simulink library "MedusaPremix"  (R2022b)
settings: Solver=VariableStepAuto  StartTime=0.0  StopTime=10.0  RelTol=1e-3
values from neighbouring files (symbols this model uses):
  PremixConfig = struct('sample_rate_in_hertz', sample_rate_in_hertz,                            'frame_size', frame_size,                            'rgain_SILENT_GAIN', rgain_SILENT_GAIN,                            'granularity', internal_granularity,                            'LR_in', LR_in, 'LR_out', LR_out,                            'CS_in', CS_in, 'CS_out', CS_out,                            'NumCenterOut' ...(+550 chars)    [MedusaPremixInit.m]
  PremixTune = MedusaPremixTuneInit(tuneFileName, headrestTuneFileName, overheadTuneFileName, MedusaParams)    [MedusaPremixInit.m]    (also in MedusaPremixTuneInit.m = load(tuneFileName))
undefined symbols (not defined in the file or in its folder): carModel, mode, MSConfig, Row
libraries: TuneVar x286, TOP x202, dspmtrx3 x146, FeaturePath x86, matrix_library x20, PooliirLib x8, Pooliir x4
(part 14 of 22)

== system MedusaPremix/PremixWithMonoSurround/Full Mixing Matrix_Center Surround/Surround Level Control/Ramper ==
  RTC Recv Trigger : Inport
  target gains (linear) : Inport  Port=2
  ramp rate : Inport  Port=3
  ramp time : Inport  Port=4
  check sequence trigger : Inport  Port=5
  Data Store Memory : DataStoreMemory  DataStoreName=Premix_Freeze_CS  ReadBeforeWriteMsg=warning  WriteAfterWriteMsg=warning  WriteAfterReadMsg=warning  ShowAdditionalParam=off  OutDataTypeStr=boolean
  Data Store Memory1 : DataStoreMemory  DataStoreName=Premix_frameCount_CS  ReadBeforeWriteMsg=warning  WriteAfterWriteMsg=warning  WriteAfterReadMsg=warning  InitialValue=zeros(MedusaPremixConfig.CS_out,MedusaPremixConfig.CS_in)  ShowAdditionalParam=off  OutDataTypeStr=int32
  Data Store Memory2 : DataStoreMemory  DataStoreName=Premix_rampCoeff_CS  ReadBeforeWriteMsg=warning  WriteAfterWriteMsg=warning  WriteAfterReadMsg=warning  InitialValue=ones(MedusaPremixConfig.CS_out,MedusaPremixConfig.CS_in)  ShowAdditionalParam=off  OutDataTypeStr=single
  check sequence : MATLAB Function  TreatAsAtomicUnit=on
  control : MATLAB Function  TreatAsAtomicUnit=on
  process : MATLAB Function  TreatAsAtomicUnit=on
  ramping done : Outport  VectorParamsAs1DForOutWhenUnconnected=off
  wires:
  target gains (linear)/1 -> control/1(target_gains_linear)
  RTC Recv Trigger/1 -> control/Trigger
  check sequence/1(done) -> ramping done/1
  check sequence trigger/1 -> check sequence/Trigger
  ramp rate/1 -> control/2(rampRate)
  ramp time/1 -> control/3(rampTime)

== system MedusaPremix/PremixWithMonoSurround/Full Mixing Matrix_Left/Fader Downmix/Fading Backward ==
  frontFadeGain : Inport
  backwardDownmixThreshold : Inport  Port=2
  backwardDownmixMax : Inport  Port=3
  Action Port : ActionPort
  Constant : Constant  OutDataTypeStr=single
  Divide : Product  Inputs=*/
  EPS : Constant  Value=eps('single')
  Max : MinMax  Function=max  Inputs=2
  Min : MinMax  Inputs=2
  Multiply : Product
  Subtract : Sum  Inputs=+-
  downmix : Outport  VectorParamsAs1DForOutWhenUnconnected=off
  wires:
  Multiply/1 -> downmix/1
  backwardDownmixMax/1 -> Multiply/2
  Subtract/1 -> Multiply/1
  Divide/1 -> Subtract/2
  Max/1 -> Divide/2
  Min/1 -> Divide/1  "minFadeGain"
  EPS/1 -> Max/2
  Constant/1 -> Subtract/1
  backwardDownmixThreshold/1 -> Max/1, Min/2
  frontFadeGain/1 -> Min/1

== system MedusaPremix/PremixWithMonoSurround/Full Mixing Matrix_Left/Fader Downmix/Fading Forward ==
  backFadeGain : Inport
  forwardDownmixThreshold : Inport  Port=2
  forwardDownmixMax : Inport  Port=3
  Action Port : ActionPort
  Constant : Constant  OutDataTypeStr=single
  Divide : Product  Inputs=*/
  EPS : Constant  Value=eps('single')
  Max : MinMax  Function=max  Inputs=2
  Min : MinMax  Inputs=2
  Multiply : Product
  Subtract : Sum  Inputs=+-
  downmix : Outport  VectorParamsAs1DForOutWhenUnconnected=off
  wires:
  Multiply/1 -> downmix/1
  forwardDownmixMax/1 -> Multiply/2
  Subtract/1 -> Multiply/1
  Divide/1 -> Subtract/2
  Max/1 -> Divide/2
  Min/1 -> Divide/1  "minFadeGain"
  EPS/1 -> Max/2
  Constant/1 -> Subtract/1
  forwardDownmixThreshold/1 -> Max/1, Min/2
  backFadeGain/1 -> Min/1

== system MedusaPremix/PremixWithMonoSurround/Full Mixing Matrix_Left/Surround Level Control/Ramper ==
  RTC Recv Trigger : Inport
  target gains (linear) : Inport  Port=2
  ramp rate : Inport  Port=3
  ramp time : Inport  Port=4
  check sequence trigger : Inport  Port=5
  Data Store Memory : DataStoreMemory  DataStoreName=Premix_Freeze_Left  ReadBeforeWriteMsg=warning  WriteAfterWriteMsg=warning  WriteAfterReadMsg=warning  ShowAdditionalParam=off  OutDataTypeStr=boolean
  Data Store Memory1 : DataStoreMemory  DataStoreName=Premix_frameCount_Left  ReadBeforeWriteMsg=warning  WriteAfterWriteMsg=warning  WriteAfterReadMsg=warning  InitialValue=zeros(MedusaPremixConfig.LR_out,MedusaPremixConfig.LR_in)  ShowAdditionalParam=off  OutDataTypeStr=int32
  Data Store Memory2 : DataStoreMemory  DataStoreName=Premix_rampCoeff_Left  ReadBeforeWriteMsg=warning  WriteAfterWriteMsg=warning  WriteAfterReadMsg=warning  InitialValue=ones(MedusaPremixConfig.LR_out,MedusaPremixConfig.LR_in)  ShowAdditionalParam=off  OutDataTypeStr=single
  check sequence : MATLAB Function  TreatAsAtomicUnit=on
  control : MATLAB Function  TreatAsAtomicUnit=on
  process : MATLAB Function  TreatAsAtomicUnit=on
  ramping done : Outport  VectorParamsAs1DForOutWhenUnconnected=off
  wires:
  target gains (linear)/1 -> control/1(target_gains_linear)
  RTC Recv Trigger/1 -> control/Trigger
  check sequence/1(done) -> ramping done/1
  check sequence trigger/1 -> check sequence/Trigger
  ramp time/1 -> control/3(rampTime)
  ramp rate/1 -> control/2(rampRate)

== system MedusaPremix/PremixWithMonoSurround/Full Mixing Matrix_Right/Fader Downmix/Fading Backward ==
  frontFadeGain : Inport
  backwardDownmixThreshold : Inport  Port=2
  backwardDownmixMax : Inport  Port=3
  Action Port : ActionPort
  Constant : Constant  OutDataTypeStr=single
  Divide : Product  Inputs=*/
  EPS : Constant  Value=eps('single')
  Max : MinMax  Function=max  Inputs=2
  Min : MinMax  Inputs=2
  Multiply : Product
  Subtract : Sum  Inputs=+-
  downmix : Outport  VectorParamsAs1DForOutWhenUnconnected=off
  wires:
  Multiply/1 -> downmix/1
  backwardDownmixMax/1 -> Multiply/2
  Subtract/1 -> Multiply/1
  Divide/1 -> Subtract/2
  Max/1 -> Divide/2
  Min/1 -> Divide/1  "minFadeGain"
  EPS/1 -> Max/2
  Constant/1 -> Subtract/1
  backwardDownmixThreshold/1 -> Max/1, Min/2
  frontFadeGain/1 -> Min/1

== system MedusaPremix/PremixWithMonoSurround/Full Mixing Matrix_Right/Fader Downmix/Fading Forward ==
  backFadeGain : Inport
  forwardDownmixThreshold : Inport  Port=2
  forwardDownmixMax : Inport  Port=3
  Action Port : ActionPort
  Constant : Constant  OutDataTypeStr=single
  Divide : Product  Inputs=*/
  EPS : Constant  Value=eps('single')
  Max : MinMax  Function=max  Inputs=2
  Min : MinMax  Inputs=2
  Multiply : Product
  Subtract : Sum  Inputs=+-
  downmix : Outport  VectorParamsAs1DForOutWhenUnconnected=off
  wires:
  Multiply/1 -> downmix/1
  forwardDownmixMax/1 -> Multiply/2
  Subtract/1 -> Multiply/1
  Divide/1 -> Subtract/2
  Max/1 -> Divide/2
  Min/1 -> Divide/1  "minFadeGain"
  EPS/1 -> Max/2
  Constant/1 -> Subtract/1
  forwardDownmixThreshold/1 -> Max/1, Min/2
  backFadeGain/1 -> Min/1

== system MedusaPremix/PremixWithMonoSurround/Full Mixing Matrix_Right/Surround Level Control/Ramper ==
  RTC Recv Trigger : Inport
  target gains (linear) : Inport  Port=2
  ramp rate : Inport  Port=3
  ramp time : Inport  Port=4
  check sequence trigger : Inport  Port=5
  Data Store Memory : DataStoreMemory  DataStoreName=Premix_Freeze_Right  ReadBeforeWriteMsg=warning  WriteAfterWriteMsg=warning  WriteAfterReadMsg=warning  ShowAdditionalParam=off  OutDataTypeStr=boolean
  Data Store Memory1 : DataStoreMemory  DataStoreName=Premix_frameCount_Right  ReadBeforeWriteMsg=warning  WriteAfterWriteMsg=warning  WriteAfterReadMsg=warning  InitialValue=zeros(MedusaPremixConfig.LR_out,MedusaPremixConfig.LR_in)  ShowAdditionalParam=off  OutDataTypeStr=int32
  Data Store Memory2 : DataStoreMemory  DataStoreName=Premix_rampCoeff_Right  ReadBeforeWriteMsg=warning  WriteAfterWriteMsg=warning  WriteAfterReadMsg=warning  InitialValue=ones(MedusaPremixConfig.LR_out,MedusaPremixConfig.LR_in)  ShowAdditionalParam=off  OutDataTypeStr=single
  check sequence : MATLAB Function  TreatAsAtomicUnit=on
  control : MATLAB Function  TreatAsAtomicUnit=on
  process : MATLAB Function  TreatAsAtomicUnit=on
  ramping done : Outport  VectorParamsAs1DForOutWhenUnconnected=off
  wires:
  target gains (linear)/1 -> control/1(target_gains_linear)
  RTC Recv Trigger/1 -> control/Trigger
  check sequence/1(done) -> ramping done/1
  check sequence trigger/1 -> check sequence/Trigger
  ramp rate/1 -> control/2(rampRate)
  ramp time/1 -> control/3(rampTime)

== system MedusaPremix/PremixWithMonoSurroundAndCae/CS Processing/Mono-Surround/Left Mixer ==
  AudioIn : Inport
  MixCoeff : Inport  Port=2
  Matrix Multiply1 : Product  Multiplication=Matrix(*)
  Transpose1 : Math  Operator=transpose  SignedPower=on
  Output : Outport  VectorParamsAs1DForOutWhenUnconnected=off
  wires:
  Transpose1/1 -> Matrix Multiply1/2
  MixCoeff/1 -> Transpose1/1
  AudioIn/1 -> Matrix Multiply1/1
  Matrix Multiply1/1 -> Output/1

== system MedusaPremix/PremixWithMonoSurroundAndCae/CS Processing/Mono-Surround/MS Tune ==
  TOP : TOP/TOP  TriggerInit=[260 -150 405 -90]  TopName=Phi  DataType=single  BankNumber=0  Role=Automatic
      settings: SourceProductName=Bose Talaria
  TOP1 : TOP/TOP  TriggerInit=[260 -70 405 -10]  TopName=CosPhi  DataType=single  BankNumber=0  Role=Automatic
      settings: SourceProductName=Bose Talaria
  TOP2 : TOP/TOP  TriggerInit=[260 10 405 70]  TopName=SinPhi  DataType=single  BankNumber=0  Role=Automatic
      settings: SourceProductName=Bose Talaria
  TranslateTrigger : TuneVar/TranslateTrigger  TriggerInit=[66 -245 104 -190]
      settings: SourceProductName=Bose Talaria
  Tune Variable : TuneVar/Tune Variable  TuneName=PhaseAngle  SpecifyMaxSize=off  VariableDim=1 (Row)  MaxSize=[1 1]  PackageName=mode  TunabilityNumber=1  MinValue=[]  MaxValue=[]  TriggerInit=[-270 -65 -100 -15]  MaskValue=MSConfig.DefaultPhaseAngle
      settings: SourceProductName=Bose Talaria
  translation : MATLAB Function  TreatAsAtomicUnit=on
  phi : Outport  VectorParamsAs1DForOutWhenUnconnected=off
  cos(phi) : Outport  Port=2  VectorParamsAs1DForOutWhenUnconnected=off
  sin(phi) : Outport  Port=3  VectorParamsAs1DForOutWhenUnconnected=off
  wires:
  TOP2/1 -> sin(phi)/1  "SinPhi"
  translation/3(sin_phi) -> TOP2/1
  TOP1/1 -> cos(phi)/1  "CosPhi"
  translation/2(cos_phi) -> TOP1/1
  Tune Variable/1 -> translation/1(PhaseAngle)  "PhaseAngle"
  TOP/1 -> phi/1  "Phi"
  TranslateTrigger/1 -> translation/Trigger
  translation/1(phi) -> TOP/1

== system MedusaPremix/PremixWithMonoSurroundAndCae/CS Processing/Mono-Surround/Right Mixer ==
  AudioIn : Inport
  MixCoeff : Inport  Port=2
  Matrix Multiply1 : Product  Multiplication=Matrix(*)
  Transpose1 : Math  Operator=transpose  SignedPower=on
  Output : Outport  VectorParamsAs1DForOutWhenUnconnected=off
  wires:
  Transpose1/1 -> Matrix Multiply1/2
  MixCoeff/1 -> Transpose1/1
  AudioIn/1 -> Matrix Multiply1/1
  Matrix Multiply1/1 -> Output/1

== system MedusaPremix/PremixWithMonoSurroundAndCae/CS Processing/Mono-Surround/SOS A ==
  AudioIn : Inport
  TuneIn : Inport  Port=2
  Hilbert SOS A : Subsystem  TreatAsAtomicUnit=on
  If : If  IfExpression=(u1==0) | (u1==180)
  Merge : Merge
  Pass-through : Subsystem  TreatAsAtomicUnit=on
  Out : Outport  VectorParamsAs1DForOutWhenUnconnected=off
  wires:
  Merge/1 -> Out/1
  Hilbert SOS A/1(Out) -> Merge/2
  Pass-through/1(Out1) -> Merge/1
  TuneIn/1 -> If/1
  If/2 -> Hilbert SOS A/Action
  If/1 -> Pass-through/Action
  AudioIn/1 -> Pass-through/1(In1), Hilbert SOS A/1(AudioIn)

== system MedusaPremix/PremixWithMonoSurroundAndCae/CS Processing/Mono-Surround/SOS B ==
  AudioIn : Inport
  TuneIn : Inport  Port=2
  Hilbert SOS B : Subsystem  TreatAsAtomicUnit=on
  If : If  IfExpression=(u1==0) | (u1==180)
  Merge : Merge
  Pass-through : Subsystem  TreatAsAtomicUnit=on
  Out : Outport  VectorParamsAs1DForOutWhenUnconnected=off
  wires:
  Merge/1 -> Out/1
  Hilbert SOS B/1(Out) -> Merge/2
  Pass-through/1(Out1) -> Merge/1
  TuneIn/1 -> If/1
  If/2 -> Hilbert SOS B/Action
  If/1 -> Pass-through/Action
  AudioIn/1 -> Pass-through/1(In1), Hilbert SOS B/1(AudioIn)

== system MedusaPremix/PremixWithMonoSurroundAndCae/Full Mixing Matrix_Center Surround/Fader Downmix/Fading Backward ==
  frontFadeGain : Inport
  backwardDownmixThreshold : Inport  Port=2
  backwardDownmixMax : Inport  Port=3
  Action Port : ActionPort
  Constant : Constant  OutDataTypeStr=single
  Divide : Product  Inputs=*/
  EPS : Constant  Value=eps('single')
  Max : MinMax  Function=max  Inputs=2
  Min : MinMax  Inputs=2
  Multiply : Product
  Subtract : Sum  Inputs=+-
  downmix : Outport  VectorParamsAs1DForOutWhenUnconnected=off
  wires:
  Multiply/1 -> downmix/1
  backwardDownmixMax/1 -> Multiply/2
  Subtract/1 -> Multiply/1
  Divide/1 -> Subtract/2
  Max/1 -> Divide/2
  Min/1 -> Divide/1  "minFadeGain"
  EPS/1 -> Max/2
  Constant/1 -> Subtract/1
  backwardDownmixThreshold/1 -> Max/1, Min/2
  frontFadeGain/1 -> Min/1

== system MedusaPremix/PremixWithMonoSurroundAndCae/Full Mixing Matrix_Center Surround/Fader Downmix/Fading Forward ==
  backFadeGain : Inport
  forwardDownmixThreshold : Inport  Port=2
  forwardDownmixMax : Inport  Port=3
  Action Port : ActionPort
  Constant : Constant  OutDataTypeStr=single
  Divide : Product  Inputs=*/
  EPS : Constant  Value=eps('single')
  Max : MinMax  Function=max  Inputs=2
  Min : MinMax  Inputs=2
  Multiply : Product
  Subtract : Sum  Inputs=+-
  downmix : Outport  VectorParamsAs1DForOutWhenUnconnected=off
  wires:
  Multiply/1 -> downmix/1
  forwardDownmixMax/1 -> Multiply/2
  Subtract/1 -> Multiply/1
  Divide/1 -> Subtract/2
  Max/1 -> Divide/2
  Min/1 -> Divide/1  "minFadeGain"
  EPS/1 -> Max/2
  Constant/1 -> Subtract/1
  forwardDownmixThreshold/1 -> Max/1, Min/2
  backFadeGain/1 -> Min/1

== system MedusaPremix/PremixWithMonoSurroundAndCae/Full Mixing Matrix_Center Surround/Surround Level Control/Ramper ==
  RTC Recv Trigger : Inport
  target gains (linear) : Inport  Port=2
  ramp rate : Inport  Port=3
  ramp time : Inport  Port=4
  check sequence trigger : Inport  Port=5
  Data Store Memory : DataStoreMemory  DataStoreName=Premix_Freeze_CS  ReadBeforeWriteMsg=warning  WriteAfterWriteMsg=warning  WriteAfterReadMsg=warning  ShowAdditionalParam=off  OutDataTypeStr=boolean
  Data Store Memory1 : DataStoreMemory  DataStoreName=Premix_frameCount_CS  ReadBeforeWriteMsg=warning  WriteAfterWriteMsg=warning  WriteAfterReadMsg=warning  InitialValue=zeros(MedusaPremixConfig.CS_out,MedusaPremixConfig.CS_in)  ShowAdditionalParam=off  OutDataTypeStr=int32
  Data Store Memory2 : DataStoreMemory  DataStoreName=Premix_rampCoeff_CS  ReadBeforeWriteMsg=warning  WriteAfterWriteMsg=warning  WriteAfterReadMsg=warning  InitialValue=ones(MedusaPremixConfig.CS_out,MedusaPremixConfig.CS_in)  ShowAdditionalParam=off  OutDataTypeStr=single
  check sequence : MATLAB Function  TreatAsAtomicUnit=on
  control : MATLAB Function  TreatAsAtomicUnit=on
  process : MATLAB Function  TreatAsAtomicUnit=on
  ramping done : Outport  VectorParamsAs1DForOutWhenUnconnected=off
  wires:
  target gains (linear)/1 -> control/1(target_gains_linear)
  RTC Recv Trigger/1 -> control/Trigger
  check sequence/1(done) -> ramping done/1
  check sequence trigger/1 -> check sequence/Trigger
  ramp rate/1 -> control/2(rampRate)
  ramp time/1 -> control/3(rampTime)

== system MedusaPremix/PremixWithMonoSurroundAndCae/Full Mixing Matrix_Left/Fader Downmix/Fading Backward ==
  frontFadeGain : Inport
  backwardDownmixThreshold : Inport  Port=2
  backwardDownmixMax : Inport  Port=3
  Action Port : ActionPort
  Constant : Constant  OutDataTypeStr=single
  Divide : Product  Inputs=*/
  EPS : Constant  Value=eps('single')
  Max : MinMax  Function=max  Inputs=2
  Min : MinMax  Inputs=2
  Multiply : Product
  Subtract : Sum  Inputs=+-
  downmix : Outport  VectorParamsAs1DForOutWhenUnconnected=off
  wires:
  Multiply/1 -> downmix/1
  backwardDownmixMax/1 -> Multiply/2
  Subtract/1 -> Multiply/1
  Divide/1 -> Subtract/2
  Max/1 -> Divide/2
  Min/1 -> Divide/1  "minFadeGain"
  EPS/1 -> Max/2
  Constant/1 -> Subtract/1
  backwardDownmixThreshold/1 -> Max/1, Min/2
  frontFadeGain/1 -> Min/1

== system MedusaPremix/PremixWithMonoSurroundAndCae/Full Mixing Matrix_Left/Fader Downmix/Fading Forward ==
  backFadeGain : Inport
  forwardDownmixThreshold : Inport  Port=2
  forwardDownmixMax : Inport  Port=3
  Action Port : ActionPort
  Constant : Constant  OutDataTypeStr=single
  Divide : Product  Inputs=*/
  EPS : Constant  Value=eps('single')
  Max : MinMax  Function=max  Inputs=2
  Min : MinMax  Inputs=2
  Multiply : Product
  Subtract : Sum  Inputs=+-
  downmix : Outport  VectorParamsAs1DForOutWhenUnconnected=off
  wires:
  Multiply/1 -> downmix/1
  forwardDownmixMax/1 -> Multiply/2
  Subtract/1 -> Multiply/1
  Divide/1 -> Subtract/2
  Max/1 -> Divide/2
  Min/1 -> Divide/1  "minFadeGain"
  EPS/1 -> Max/2
  Constant/1 -> Subtract/1
  forwardDownmixThreshold/1 -> Max/1, Min/2
  backFadeGain/1 -> Min/1

== system MedusaPremix/PremixWithMonoSurroundAndCae/Full Mixing Matrix_Left/Surround Level Control/Ramper ==
  RTC Recv Trigger : Inport
  target gains (linear) : Inport  Port=2
  ramp rate : Inport  Port=3
  ramp time : Inport  Port=4
  check sequence trigger : Inport  Port=5
  Data Store Memory : DataStoreMemory  DataStoreName=Premix_Freeze_Left  ReadBeforeWriteMsg=warning  WriteAfterWriteMsg=warning  WriteAfterReadMsg=warning  ShowAdditionalParam=off  OutDataTypeStr=boolean
  Data Store Memory1 : DataStoreMemory  DataStoreName=Premix_frameCount_Left  ReadBeforeWriteMsg=warning  WriteAfterWriteMsg=warning  WriteAfterReadMsg=warning  InitialValue=zeros(MedusaPremixConfig.LR_out,MedusaPremixConfig.LR_in)  ShowAdditionalParam=off  OutDataTypeStr=int32
  Data Store Memory2 : DataStoreMemory  DataStoreName=Premix_rampCoeff_Left  ReadBeforeWriteMsg=warning  WriteAfterWriteMsg=warning  WriteAfterReadMsg=warning  InitialValue=ones(MedusaPremixConfig.LR_out,MedusaPremixConfig.LR_in)  ShowAdditionalParam=off  OutDataTypeStr=single
  check sequence : MATLAB Function  TreatAsAtomicUnit=on
  control : MATLAB Function  TreatAsAtomicUnit=on
  process : MATLAB Function  TreatAsAtomicUnit=on
  ramping done : Outport  VectorParamsAs1DForOutWhenUnconnected=off
  wires:
  target gains (linear)/1 -> control/1(target_gains_linear)
  RTC Recv Trigger/1 -> control/Trigger
  check sequence/1(done) -> ramping done/1
  check sequence trigger/1 -> check sequence/Trigger
  ramp time/1 -> control/3(rampTime)
  ramp rate/1 -> control/2(rampRate)

== system MedusaPremix/PremixWithMonoSurroundAndCae/Full Mixing Matrix_Right/Fader Downmix/Fading Backward ==
  frontFadeGain : Inport
  backwardDownmixThreshold : Inport  Port=2
  backwardDownmixMax : Inport  Port=3
  Action Port : ActionPort
  Constant : Constant  OutDataTypeStr=single
  Divide : Product  Inputs=*/
  EPS : Constant  Value=eps('single')
  Max : MinMax  Function=max  Inputs=2
  Min : MinMax  Inputs=2
  Multiply : Product
  Subtract : Sum  Inputs=+-
  downmix : Outport  VectorParamsAs1DForOutWhenUnconnected=off
  wires:
  Multiply/1 -> downmix/1
  backwardDownmixMax/1 -> Multiply/2
  Subtract/1 -> Multiply/1
  Divide/1 -> Subtract/2
  Max/1 -> Divide/2
  Min/1 -> Divide/1  "minFadeGain"
  EPS/1 -> Max/2
  Constant/1 -> Subtract/1
  backwardDownmixThreshold/1 -> Max/1, Min/2
  frontFadeGain/1 -> Min/1

== system MedusaPremix/PremixWithMonoSurroundAndCae/Full Mixing Matrix_Right/Fader Downmix/Fading Forward ==
  backFadeGain : Inport
  forwardDownmixThreshold : Inport  Port=2
  forwardDownmixMax : Inport  Port=3
  Action Port : ActionPort
  Constant : Constant  OutDataTypeStr=single
  Divide : Product  Inputs=*/
  EPS : Constant  Value=eps('single')
  Max : MinMax  Function=max  Inputs=2
  Min : MinMax  Inputs=2
  Multiply : Product
  Subtract : Sum  Inputs=+-
  downmix : Outport  VectorParamsAs1DForOutWhenUnconnected=off
  wires:
  Multiply/1 -> downmix/1
  forwardDownmixMax/1 -> Multiply/2
  Subtract/1 -> Multiply/1
  Divide/1 -> Subtract/2
  Max/1 -> Divide/2
  Min/1 -> Divide/1  "minFadeGain"
  EPS/1 -> Max/2
  Constant/1 -> Subtract/1
  forwardDownmixThreshold/1 -> Max/1, Min/2
  backFadeGain/1 -> Min/1

== system MedusaPremix/PremixWithMonoSurroundAndCae/Full Mixing Matrix_Right/Surround Level Control/Ramper ==
  RTC Recv Trigger : Inport
  target gains (linear) : Inport  Port=2
  ramp rate : Inport  Port=3
  ramp time : Inport  Port=4
  check sequence trigger : Inport  Port=5
  Data Store Memory : DataStoreMemory  DataStoreName=Premix_Freeze_Right  ReadBeforeWriteMsg=warning  WriteAfterWriteMsg=warning  WriteAfterReadMsg=warning  ShowAdditionalParam=off  OutDataTypeStr=boolean
  Data Store Memory1 : DataStoreMemory  DataStoreName=Premix_frameCount_Right  ReadBeforeWriteMsg=warning  WriteAfterWriteMsg=warning  WriteAfterReadMsg=warning  InitialValue=zeros(MedusaPremixConfig.LR_out,MedusaPremixConfig.LR_in)  ShowAdditionalParam=off  OutDataTypeStr=int32
  Data Store Memory2 : DataStoreMemory  DataStoreName=Premix_rampCoeff_Right  ReadBeforeWriteMsg=warning  WriteAfterWriteMsg=warning  WriteAfterReadMsg=warning  InitialValue=ones(MedusaPremixConfig.LR_out,MedusaPremixConfig.LR_in)  ShowAdditionalParam=off  OutDataTypeStr=single
  check sequence : MATLAB Function  TreatAsAtomicUnit=on
  control : MATLAB Function  TreatAsAtomicUnit=on
  process : MATLAB Function  TreatAsAtomicUnit=on
  ramping done : Outport  VectorParamsAs1DForOutWhenUnconnected=off
  wires:
  target gains (linear)/1 -> control/1(target_gains_linear)
  RTC Recv Trigger/1 -> control/Trigger
  check sequence/1(done) -> ramping done/1
  check sequence trigger/1 -> check sequence/Trigger
  ramp rate/1 -> control/2(rampRate)
  ramp time/1 -> control/3(rampTime)

== system MedusaPremix/PremixWithMonoSurroundAndCaeWithFadeRamper/CS Processing/Mono-Surround/Left Mixer ==
  AudioIn : Inport
  MixCoeff : Inport  Port=2
  Matrix Multiply1 : Product  Multiplication=Matrix(*)
  Transpose1 : Math  Operator=transpose  SignedPower=on
  Output : Outport  VectorParamsAs1DForOutWhenUnconnected=off
  wires:
  Matrix Multiply1/1 -> Output/1
  AudioIn/1 -> Matrix Multiply1/1
  MixCoeff/1 -> Transpose1/1
  Transpose1/1 -> Matrix Multiply1/2

== system MedusaPremix/PremixWithMonoSurroundAndCaeWithFadeRamper/CS Processing/Mono-Surround/Right Mixer ==
  AudioIn : Inport
  MixCoeff : Inport  Port=2
  Matrix Multiply1 : Product  Multiplication=Matrix(*)
  Transpose1 : Math  Operator=transpose  SignedPower=on
  Output : Outport  VectorParamsAs1DForOutWhenUnconnected=off
  wires:
  Matrix Multiply1/1 -> Output/1
  AudioIn/1 -> Matrix Multiply1/1
  MixCoeff/1 -> Transpose1/1
  Transpose1/1 -> Matrix Multiply1/2

== system MedusaPremix/PremixWithMonoSurroundAndCaeWithFadeRamper/CS Processing/Mono-Surround/SOS A ==
  AudioIn : Inport
  TuneIn : Inport  Port=2
  Hilbert SOS A : Subsystem  TreatAsAtomicUnit=on
  If : If  IfExpression=(u1==0) | (u1==180)
  Merge : Merge
  Pass-through : Subsystem  TreatAsAtomicUnit=on
  Output : Outport  VectorParamsAs1DForOutWhenUnconnected=off
  wires:
  AudioIn/1 -> Hilbert SOS A/1(AudioIn), Pass-through/1(In1)
  If/1 -> Pass-through/Action
  If/2 -> Hilbert SOS A/Action
  TuneIn/1 -> If/1
  Pass-through/1(Out1) -> Merge/1
  Merge/1 -> Output/1
  Hilbert SOS A/1(Out) -> Merge/2

== system MedusaPremix/PremixWithMonoSurroundAndCaeWithFadeRamper/CS Processing/Mono-Surround/SOS B ==
  AudioIn : Inport
  TuneIn : Inport  Port=2
  Hilbert SOS B : Subsystem  TreatAsAtomicUnit=on
  If : If  IfExpression=(u1==0) | (u1==180)
  Merge : Merge
  Pass-through : Subsystem  TreatAsAtomicUnit=on
  Out : Outport  VectorParamsAs1DForOutWhenUnconnected=off
  wires:
  AudioIn/1 -> Hilbert SOS B/1(AudioIn), Pass-through/1(In1)
  If/1 -> Pass-through/Action
  If/2 -> Hilbert SOS B/Action
  TuneIn/1 -> If/1
  Pass-through/1(Out1) -> Merge/1
  Merge/1 -> Out/1
  Hilbert SOS B/1(Out) -> Merge/2

== system MedusaPremix/PremixWithMonoSurroundAndCaeWithFadeRamper/Full Mixing Matrix_Center Surround/Fader Downmix/Fading Backward ==
  frontFadeGain : Inport
  backwardDownmixThreshold : Inport  Port=2
  backwardDownmixMax : Inport  Port=3
  Action Port : ActionPort
  Constant : Constant  OutDataTypeStr=single
  Divide : Product  Inputs=*/
  EPS : Constant  Value=eps('single')
  Max : MinMax  Function=max  Inputs=2
  Min : MinMax  Inputs=2
  Multiply : Product
  Subtract : Sum  Inputs=+-
  downmix : Outport  VectorParamsAs1DForOutWhenUnconnected=off
  wires:
  frontFadeGain/1 -> Min/1
  backwardDownmixThreshold/1 -> Min/2, Max/1
  Constant/1 -> Subtract/1
  EPS/1 -> Max/2
  Min/1 -> Divide/1  "minFadeGain"
  Max/1 -> Divide/2
  Divide/1 -> Subtract/2
  Subtract/1 -> Multiply/1
  backwardDownmixMax/1 -> Multiply/2
  Multiply/1 -> downmix/1

== system MedusaPremix/PremixWithMonoSurroundAndCaeWithFadeRamper/Full Mixing Matrix_Center Surround/Fader Downmix/Fading Forward ==
  backFadeGain : Inport
  forwardDownmixThreshold : Inport  Port=2
  forwardDownmixMax : Inport  Port=3
  Action Port : ActionPort
  Constant : Constant  OutDataTypeStr=single
  Divide : Product  Inputs=*/
  EPS : Constant  Value=eps('single')
  Max : MinMax  Function=max  Inputs=2
  Min : MinMax  Inputs=2
  Multiply : Product
  Subtract : Sum  Inputs=+-
  downmix : Outport  VectorParamsAs1DForOutWhenUnconnected=off
  wires:
  backFadeGain/1 -> Min/1
  forwardDownmixThreshold/1 -> Min/2, Max/1
  Constant/1 -> Subtract/1
  EPS/1 -> Max/2
  Min/1 -> Divide/1  "minFadeGain"
  Max/1 -> Divide/2
  Divide/1 -> Subtract/2
  Subtract/1 -> Multiply/1
  forwardDownmixMax/1 -> Multiply/2
  Multiply/1 -> downmix/1

== system MedusaPremix/PremixWithMonoSurroundAndCaeWithFadeRamper/Full Mixing Matrix_Left/Fader Downmix/Fading Backward ==
  frontFadeGain : Inport
  backwardDownmixThreshold : Inport  Port=2
  backwardDownmixMax : Inport  Port=3
  Action Port : ActionPort
  Constant : Constant  OutDataTypeStr=single
  Divide : Product  Inputs=*/
  EPS : Constant  Value=eps('single')
  Max : MinMax  Function=max  Inputs=2
  Min : MinMax  Inputs=2
  Multiply : Product
  Subtract : Sum  Inputs=+-
  downmix : Outport  VectorParamsAs1DForOutWhenUnconnected=off
  wires:
  frontFadeGain/1 -> Min/1
  backwardDownmixThreshold/1 -> Min/2, Max/1
  Constant/1 -> Subtract/1
  EPS/1 -> Max/2
  Min/1 -> Divide/1  "minFadeGain"
  Max/1 -> Divide/2
  Divide/1 -> Subtract/2
  Subtract/1 -> Multiply/1
  backwardDownmixMax/1 -> Multiply/2
  Multiply/1 -> downmix/1

== system MedusaPremix/PremixWithMonoSurroundAndCaeWithFadeRamper/Full Mixing Matrix_Left/Fader Downmix/Fading Forward ==
  backFadeGain : Inport
  forwardDownmixThreshold : Inport  Port=2
  forwardDownmixMax : Inport  Port=3
  Action Port : ActionPort
  Constant : Constant  OutDataTypeStr=single
  Divide : Product  Inputs=*/
  EPS : Constant  Value=eps('single')
  Max : MinMax  Function=max  Inputs=2
  Min : MinMax  Inputs=2
  Multiply : Product
  Subtract : Sum  Inputs=+-
  downmix : Outport  VectorParamsAs1DForOutWhenUnconnected=off
  wires:
  backFadeGain/1 -> Min/1
  forwardDownmixThreshold/1 -> Min/2, Max/1
  Constant/1 -> Subtract/1
  EPS/1 -> Max/2
  Min/1 -> Divide/1  "minFadeGain"
  Max/1 -> Divide/2
  Divide/1 -> Subtract/2
  Subtract/1 -> Multiply/1
  forwardDownmixMax/1 -> Multiply/2
  Multiply/1 -> downmix/1

== system MedusaPremix/PremixWithMonoSurroundAndCaeWithFadeRamper/Full Mixing Matrix_Right/Fader Downmix/Fading Backward ==
  frontFadeGain : Inport
  backwardDownmixThreshold : Inport  Port=2
  backwardDownmixMax : Inport  Port=3
  Action Port : ActionPort
  Constant : Constant  OutDataTypeStr=single
  Divide : Product  Inputs=*/
  EPS : Constant  Value=eps('single')
  Max : MinMax  Function=max  Inputs=2
  Min : MinMax  Inputs=2
  Multiply : Product
  Subtract : Sum  Inputs=+-
  downmix : Outport  VectorParamsAs1DForOutWhenUnconnected=off
  wires:
  frontFadeGain/1 -> Min/1
  backwardDownmixThreshold/1 -> Min/2, Max/1
  Constant/1 -> Subtract/1
  EPS/1 -> Max/2
  Min/1 -> Divide/1  "minFadeGain"
  Max/1 -> Divide/2
  Divide/1 -> Subtract/2
  Subtract/1 -> Multiply/1
  backwardDownmixMax/1 -> Multiply/2
  Multiply/1 -> downmix/1

== system MedusaPremix/PremixWithMonoSurroundAndCaeWithFadeRamper/Full Mixing Matrix_Right/Fader Downmix/Fading Forward ==
  backFadeGain : Inport
  forwardDownmixThreshold : Inport  Port=2
  forwardDownmixMax : Inport  Port=3
  Action Port : ActionPort
  Constant : Constant  OutDataTypeStr=single
  Divide : Product  Inputs=*/
  EPS : Constant  Value=eps('single')
  Max : MinMax  Function=max  Inputs=2
  Min : MinMax  Inputs=2
  Multiply : Product
  Subtract : Sum  Inputs=+-
  downmix : Outport  VectorParamsAs1DForOutWhenUnconnected=off
  wires:
  backFadeGain/1 -> Min/1
  forwardDownmixThreshold/1 -> Min/2, Max/1
  Constant/1 -> Subtract/1
  EPS/1 -> Max/2
  Min/1 -> Divide/1  "minFadeGain"
  Max/1 -> Divide/2
  Divide/1 -> Subtract/2
  Subtract/1 -> Multiply/1
  forwardDownmixMax/1 -> Multiply/2
  Multiply/1 -> downmix/1

== system MedusaPremix/Premix51WithMonoSurround/CS Processing/Mono-Surround/SOS A/Hilbert SOS A ==
  AudioIn : Inport
  Action Port : ActionPort
  Constant : Constant  Value=MSConfig.hilbPairNumStagesA  OutDataTypeStr=uint32  SampleTime=-1
  Constant1 : Constant  Value=MSConfig.hilbPairCoeffsA  OutDataTypeStr=single  SampleTime=-1
  Pooliir with no TuneTOP : Pooliir/Pooliir with no TuneTOP  maxNumStages=MSConfig.maxNumStages
  Out : Outport  VectorParamsAs1DForOutWhenUnconnected=off
  wires:
  AudioIn/1 -> Pooliir with no TuneTOP/1
  Pooliir with no TuneTOP/1 -> Out/1
  Constant/1 -> Pooliir with no TuneTOP/2
  Constant1/1 -> Pooliir with no TuneTOP/3

== system MedusaPremix/Premix51WithMonoSurround/CS Processing/Mono-Surround/SOS A/Pass-through ==
  In1 : Inport
  Action Port : ActionPort
  Out1 : Outport  VectorParamsAs1DForOutWhenUnconnected=off
  wires:
  In1/1 -> Out1/1

== system MedusaPremix/Premix51WithMonoSurround/CS Processing/Mono-Surround/SOS B/Hilbert SOS B ==
  AudioIn : Inport
  Action Port : ActionPort
  Constant : Constant  Value=MSConfig.hilbPairNumStagesB  OutDataTypeStr=uint32  SampleTime=-1
  Constant1 : Constant  Value=MSConfig.hilbPairCoeffsB  OutDataTypeStr=single  SampleTime=-1
  Pooliir with no TuneTOP : Pooliir/Pooliir with no TuneTOP  maxNumStages=MSConfig.maxNumStages
  Out : Outport  VectorParamsAs1DForOutWhenUnconnected=off
  wires:
  AudioIn/1 -> Pooliir with no TuneTOP/1
  Pooliir with no TuneTOP/1 -> Out/1
  Constant/1 -> Pooliir with no TuneTOP/2
  Constant1/1 -> Pooliir with no TuneTOP/3

== system MedusaPremix/Premix51WithMonoSurround/CS Processing/Mono-Surround/SOS B/Pass-through ==
  In1 : Inport
  Action Port : ActionPort
  Out1 : Outport  VectorParamsAs1DForOutWhenUnconnected=off
  wires:
  In1/1 -> Out1/1

== system MedusaPremix/Premix51WithMonoSurroundAndCae/CS Processing/Mono-Surround/SOS A/Hilbert SOS A ==
  AudioIn : Inport
  Action Port : ActionPort
  Constant : Constant  Value=MSConfig.hilbPairNumStagesA  OutDataTypeStr=uint32  SampleTime=-1
  Constant1 : Constant  Value=MSConfig.hilbPairCoeffsA  OutDataTypeStr=single  SampleTime=-1
  Pooliir with no TuneTOP : PooliirLib/Pooliir with no TuneTOP  maxNumStages=MSConfig.maxNumStages  variantType=MSConfig.variant
  Out : Outport  VectorParamsAs1DForOutWhenUnconnected=off
  wires:
  AudioIn/1 -> Pooliir with no TuneTOP/1
  Pooliir with no TuneTOP/1 -> Out/1
  Constant/1 -> Pooliir with no TuneTOP/2
  Constant1/1 -> Pooliir with no TuneTOP/4, Pooliir with no TuneTOP/3

== system MedusaPremix/Premix51WithMonoSurroundAndCae/CS Processing/Mono-Surround/SOS A/Pass-through ==
  In1 : Inport
  Action Port : ActionPort
  Out1 : Outport  VectorParamsAs1DForOutWhenUnconnected=off
  wires:
  In1/1 -> Out1/1

== system MedusaPremix/Premix51WithMonoSurroundAndCae/CS Processing/Mono-Surround/SOS B/Hilbert SOS B ==
  AudioIn : Inport
  Action Port : ActionPort
  Constant : Constant  Value=MSConfig.hilbPairNumStagesB  OutDataTypeStr=uint32  SampleTime=-1
  Constant1 : Constant  Value=MSConfig.hilbPairCoeffsB  OutDataTypeStr=single  SampleTime=-1
  Pooliir with no TuneTOP : PooliirLib/Pooliir with no TuneTOP  maxNumStages=MSConfig.maxNumStages  variantType=MSConfig.variant
  Out : Outport  VectorParamsAs1DForOutWhenUnconnected=off
  wires:
  AudioIn/1 -> Pooliir with no TuneTOP/1
  Pooliir with no TuneTOP/1 -> Out/1
  Constant/1 -> Pooliir with no TuneTOP/2
  Constant1/1 -> Pooliir with no TuneTOP/4, Pooliir with no TuneTOP/3

== system MedusaPremix/Premix51WithMonoSurroundAndCae/CS Processing/Mono-Surround/SOS B/Pass-through ==
  In1 : Inport
  Action Port : ActionPort
  Out1 : Outport  VectorParamsAs1DForOutWhenUnconnected=off
  wires:
  In1/1 -> Out1/1

== system MedusaPremix/Premix51WithMonoSurroundAndCaeWithFadeRamper/CS Processing/Mono-Surround/SOS A/Hilbert SOS A ==
  AudioIn : Inport
  Action Port : ActionPort
  Constant : Constant  Value=MSConfig.hilbPairNumStagesA  OutDataTypeStr=uint32  SampleTime=-1
  Constant1 : Constant  Value=MSConfig.hilbPairCoeffsA  OutDataTypeStr=single  SampleTime=-1
  Pooliir with no TuneTOP : PooliirLib/Pooliir with no TuneTOP  maxNumStages=MSConfig.maxNumStages  variantType=MSConfig.variant
  Out : Outport  VectorParamsAs1DForOutWhenUnconnected=off
  wires:
  AudioIn/1 -> Pooliir with no TuneTOP/1
  Pooliir with no TuneTOP/1 -> Out/1
  Constant/1 -> Pooliir with no TuneTOP/2
  Constant1/1 -> Pooliir with no TuneTOP/4, Pooliir with no TuneTOP/3

== system MedusaPremix/Premix51WithMonoSurroundAndCaeWithFadeRamper/CS Processing/Mono-Surround/SOS A/Pass-through ==
  In1 : Inport
  Action Port : ActionPort
  Out1 : Outport  VectorParamsAs1DForOutWhenUnconnected=off
  wires:
  In1/1 -> Out1/1

== system MedusaPremix/Premix51WithMonoSurroundAndCaeWithFadeRamper/CS Processing/Mono-Surround/SOS B/Hilbert SOS B ==
  AudioIn : Inport
  Action Port : ActionPort
  Constant : Constant  Value=MSConfig.hilbPairNumStagesB  OutDataTypeStr=uint32  SampleTime=-1
  Constant1 : Constant  Value=MSConfig.hilbPairCoeffsB  OutDataTypeStr=single  SampleTime=-1
  Pooliir with no TuneTOP : PooliirLib/Pooliir with no TuneTOP  maxNumStages=MSConfig.maxNumStages  variantType=MSConfig.variant
  Out : Outport  VectorParamsAs1DForOutWhenUnconnected=off
  wires:
  AudioIn/1 -> Pooliir with no TuneTOP/1
  Pooliir with no TuneTOP/1 -> Out/1
  Constant/1 -> Pooliir with no TuneTOP/2
  Constant1/1 -> Pooliir with no TuneTOP/4, Pooliir with no TuneTOP/3

== system MedusaPremix/Premix51WithMonoSurroundAndCaeWithFadeRamper/CS Processing/Mono-Surround/SOS B/Pass-through ==
  In1 : Inport
  Action Port : ActionPort
  Out1 : Outport  VectorParamsAs1DForOutWhenUnconnected=off
  wires:
  In1/1 -> Out1/1

== system MedusaPremix/PremixWithMonoSurround/CS Processing/Mono-Surround/SOS A/Hilbert SOS A ==
  AudioIn : Inport
  Action Port : ActionPort
  Constant : Constant  Value=MSConfig.hilbPairNumStagesA  OutDataTypeStr=uint32  SampleTime=-1
  Constant1 : Constant  Value=MSConfig.hilbPairCoeffsA  OutDataTypeStr=single  SampleTime=-1
  Pooliir with no TuneTOP : Pooliir/Pooliir with no TuneTOP  maxNumStages=MSConfig.maxNumStages
  Out : Outport  VectorParamsAs1DForOutWhenUnconnected=off
  wires:
  AudioIn/1 -> Pooliir with no TuneTOP/1
  Pooliir with no TuneTOP/1 -> Out/1
  Constant/1 -> Pooliir with no TuneTOP/2
  Constant1/1 -> Pooliir with no TuneTOP/3

== system MedusaPremix/PremixWithMonoSurround/CS Processing/Mono-Surround/SOS A/Pass-through ==
  In1 : Inport
  Action Port : ActionPort
  Out1 : Outport  VectorParamsAs1DForOutWhenUnconnected=off
  wires:
  In1/1 -> Out1/1

== system MedusaPremix/PremixWithMonoSurround/CS Processing/Mono-Surround/SOS B/Hilbert SOS B ==
  AudioIn : Inport
  Action Port : ActionPort
  Constant : Constant  Value=MSConfig.hilbPairNumStagesB  OutDataTypeStr=uint32  SampleTime=-1
  Constant1 : Constant  Value=MSConfig.hilbPairCoeffsB  OutDataTypeStr=single  SampleTime=-1
  Pooliir with no TuneTOP : Pooliir/Pooliir with no TuneTOP  maxNumStages=MSConfig.maxNumStages
  Out : Outport  VectorParamsAs1DForOutWhenUnconnected=off
  wires:
  AudioIn/1 -> Pooliir with no TuneTOP/1
  Pooliir with no TuneTOP/1 -> Out/1
  Constant/1 -> Pooliir with no TuneTOP/2
  Constant1/1 -> Pooliir with no TuneTOP/3

== system MedusaPremix/PremixWithMonoSurround/CS Processing/Mono-Surround/SOS B/Pass-through ==
  In1 : Inport
  Action Port : ActionPort
  Out1 : Outport  VectorParamsAs1DForOutWhenUnconnected=off
  wires:
  In1/1 -> Out1/1

== system MedusaPremix/PremixWithMonoSurroundAndCae/CS Processing/Mono-Surround/SOS A/Hilbert SOS A ==
  AudioIn : Inport
  Action Port : ActionPort
  Constant : Constant  Value=MSConfig.hilbPairNumStagesA  OutDataTypeStr=uint32  SampleTime=-1
  Constant1 : Constant  Value=MSConfig.hilbPairCoeffsA  OutDataTypeStr=single  SampleTime=-1
  Pooliir with no TuneTOP : PooliirLib/Pooliir with no TuneTOP  maxNumStages=MSConfig.maxNumStages  variantType=MSConfig.variant
  Out : Outport  VectorParamsAs1DForOutWhenUnconnected=off
  wires:
  Constant1/1 -> Pooliir with no TuneTOP/4, Pooliir with no TuneTOP/3
  Constant/1 -> Pooliir with no TuneTOP/2
  Pooliir with no TuneTOP/1 -> Out/1
  AudioIn/1 -> Pooliir with no TuneTOP/1

== system MedusaPremix/PremixWithMonoSurroundAndCae/CS Processing/Mono-Surround/SOS A/Pass-through ==
  In1 : Inport
  Action Port : ActionPort
  Out1 : Outport  VectorParamsAs1DForOutWhenUnconnected=off
  wires:
  In1/1 -> Out1/1

== system MedusaPremix/PremixWithMonoSurroundAndCae/CS Processing/Mono-Surround/SOS B/Hilbert SOS B ==
  AudioIn : Inport
  Action Port : ActionPort
  Constant : Constant  Value=MSConfig.hilbPairNumStagesB  OutDataTypeStr=uint32  SampleTime=-1
  Constant1 : Constant  Value=MSConfig.hilbPairCoeffsB  OutDataTypeStr=single  SampleTime=-1
  Pooliir with no TuneTOP : PooliirLib/Pooliir with no TuneTOP  maxNumStages=MSConfig.maxNumStages  variantType=MSConfig.variant
  Out : Outport  VectorParamsAs1DForOutWhenUnconnected=off
  wires:
  Constant1/1 -> Pooliir with no TuneTOP/4, Pooliir with no TuneTOP/3
  Constant/1 -> Pooliir with no TuneTOP/2
  Pooliir with no TuneTOP/1 -> Out/1
  AudioIn/1 -> Pooliir with no TuneTOP/1

== system MedusaPremix/PremixWithMonoSurroundAndCae/CS Processing/Mono-Surround/SOS B/Pass-through ==
  In1 : Inport
  Action Port : ActionPort
  Out1 : Outport  VectorParamsAs1DForOutWhenUnconnected=off
  wires:
  In1/1 -> Out1/1

== system MedusaPremix/PremixWithMonoSurroundAndCaeWithFadeRamper/CS Processing/Mono-Surround/SOS A/Hilbert SOS A ==
  AudioIn : Inport
  Action Port : ActionPort
  Constant : Constant  Value=MSConfig.hilbPairNumStagesA  OutDataTypeStr=uint32  SampleTime=-1
  Constant1 : Constant  Value=MSConfig.hilbPairCoeffsA  OutDataTypeStr=single  SampleTime=-1
  Pooliir with no TuneTOP : PooliirLib/Pooliir with no TuneTOP  maxNumStages=MSConfig.maxNumStages  alias='MedusaPremixCSsosA'  variantType=MSConfig.variant
  Out : Outport  VectorParamsAs1DForOutWhenUnconnected=off
  wires:
  AudioIn/1 -> Pooliir with no TuneTOP/1
  Constant/1 -> Pooliir with no TuneTOP/2
  Constant1/1 -> Pooliir with no TuneTOP/3
  Pooliir with no TuneTOP/1 -> Out/1

== system MedusaPremix/PremixWithMonoSurroundAndCaeWithFadeRamper/CS Processing/Mono-Surround/SOS A/Pass-through ==
  In1 : Inport
  Action Port : ActionPort
  Out1 : Outport  VectorParamsAs1DForOutWhenUnconnected=off
  wires:
  In1/1 -> Out1/1

== system MedusaPremix/PremixWithMonoSurroundAndCaeWithFadeRamper/CS Processing/Mono-Surround/SOS B/Hilbert SOS B ==
  AudioIn : Inport
  Action Port : ActionPort
  Constant : Constant  Value=MSConfig.hilbPairNumStagesB  OutDataTypeStr=uint32  SampleTime=-1
  Constant1 : Constant  Value=MSConfig.hilbPairCoeffsB  OutDataTypeStr=single  SampleTime=-1
  Pooliir with no TuneTOP : PooliirLib/Pooliir with no TuneTOP  maxNumStages=MSConfig.maxNumStages  alias='MedusaPremixCSsosB'  variantType=MSConfig.variant
  Out : Outport  VectorParamsAs1DForOutWhenUnconnected=off
  wires:
  AudioIn/1 -> Pooliir with no TuneTOP/1
  Pooliir with no TuneTOP/1 -> Out/1
  Constant/1 -> Pooliir with no TuneTOP/2
  Constant1/1 -> Pooliir with no TuneTOP/3

== system MedusaPremix/PremixWithMonoSurroundAndCaeWithFadeRamper/CS Processing/Mono-Surround/SOS B/Pass-through ==
  In1 : Inport
  Action Port : ActionPort
  Out1 : Outport  VectorParamsAs1DForOutWhenUnconnected=off
  wires:
  In1/1 -> Out1/1

== matlab function MedusaPremix/PremixWithMonoSurround/Full Mixing Matrix_Right/Surround Level Control/Ramper/process ==
  data: Premix_Freeze_Right data_store_memory; Premix_currentGain_Right data_store_memory; Premix_targetGain_Right data_store_memory; Premix_frameCount_Right data_store_memory; Premix_rampCoeff_Right data_store_memory
function process
%#codegen

    global Premix_Freeze_Right;
    global Premix_currentGain_Right;
    global Premix_targetGain_Right;
    global Premix_frameCount_Right;
    global Premix_rampCoeff_Right;

    for i = 1:numel(Premix_currentGain_Right)
        if (Premix_Freeze_Right(1) == false)
            if (Premix_frameCount_Right(i) == 0)
                % The ramp is finished. Stop ramping and SNAP to the target
                 Premix_currentGain_Right(i) = Premix_targetGain_Right(i);
            else
                % The ramp is *NOT* frozen or done: gain is moving
                Premix_currentGain_Right(i) = Premix_currentGain_Right(i)*Premix_rampCoeff_Right(i);
                Premix_frameCount_Right(i) = Premix_frameCount_Right(i) - 1;
            end
        end
    end

end

== matlab function MedusaPremix/PremixWithMonoSurround/Full Mixing Matrix_Right/Surround Level Control/Target Gain Computation ==
  data: minGain_Right input; detentGain_Right input; maxGain_Right input; interpolation_method input; surr_level input; gain_out output; MedusaPremixConfig parameter
  events: trigger input FUNCTION_CALL_EVENT
function gain_out = generate_gain(minGain_Right, detentGain_Right, maxGain_Right, interpolation_method, surr_level, MedusaPremixConfig)
% #codegen
    
    % Extracting the surround level indices correponding to the anchor
    % points from Premix Config
    midIndex = ceil(length(MedusaPremixConfig.granularity)/2);
    min_level = MedusaPremixConfig.granularity(1);
    detent_level = MedusaPremixConfig.granularity(midIndex);
    max_level = MedusaPremixConfig.granularity(end);

    % Computing the 'surround' part of mixing gains depending on the surround
    % level index; The other part of mixing gain comes from 'fade downmix'
    switch surr_level
        case min_level
            targetGain = minGain_Right;         % when surround index corresponds to 'min' anchor point
        case detent_level
            targetGain = detentGain_Right;      % when surround index corresponds to 'detent' anchor point
        case max_level
            targetGain = maxGain_Right;         % when surround index corresponds to 'max' anchor point
        otherwise
            position = (single(surr_level) - min_level)/(max_level - min_level);            % when surround index lies in between the anchor points
            if (interpolation_method(1) == 0)
                targetGain = (maxGain_Right - minGain_Right)*position + minGain_Right;      % Linear Interpolation
            else
                minGain_dB = 20*log10(max(minGain_Right, eps('single')));
                maxGain_dB = 20*log10(max(maxGain_Right, eps('single')));
                targetGain_dB = (maxGain_dB - minGain_dB)*position + minGain_dB;
                targetGain = 10.^(targetGain_dB/20);                                        % dB-Linear Interpolation
            end
    end
    
    gain_out = targetGain;
end

== matlab function MedusaPremix/Premix/Full Mixing Matrix_Center Surround/Surround Level Control/Ramper/check sequence ==
  data: done output; Premix_currentGain_CS data_store_memory; Premix_targetGain_CS data_store_memory
  events: trigger input FUNCTION_CALL_EVENT
function done = GetCompletedSequence
% #codegen

    global Premix_currentGain_CS;
    global Premix_targetGain_CS;

    % Assume the work is complete until proven otherwise
    done = true;

    for i=1:numel(Premix_targetGain_CS)
       if (Premix_targetGain_CS(i) ~= Premix_currentGain_CS(i))
           done = false; % just proved otherwise
           break;
       end
    end

end

== matlab function MedusaPremix/PremixWithMonoSurround/SLC Tuning/Detent Level CS/Trivial Translation ==
  data: TOP output; detentGain_CS input; MedusaPremixConfig parameter
  events: trigger input FUNCTION_CALL_EVENT
function TOP  = fcn(detentGain_CS, MedusaPremixConfig)
%#codegen
% Checks if the parameter satisfies dimensionality requirements
if(detentGain_CS.Size(1) ~= MedusaPremixConfig.CS_out || detentGain_CS.Size(2) ~= MedusaPremixConfig.CS_in)
    TranslateError('The parameter ''medusa_premix_cs_detent'' must be a matrix consisting of %d rows and %d columns.', MedusaPremixConfig.CS_out, MedusaPremixConfig.CS_in);
end

% Checks if the parameter values follow bound requirements
checkValues = (detentGain_CS.Value < 0);    
if(sum(sum(checkValues)))       % Results in 0 if all values in the matrix respect the bound requirements
    TranslateError('The weights in ''medusa_premix_cs_detent'' must be greater than or equal to 0.');
end

TOP = detentGain_CS.Value;

end

== matlab function MedusaPremix/PremixWithMonoSurround/SLC Tuning/Detent Level Left/Trivial Translation ==
  data: TOP output; detentGain_Left input; MedusaPremixConfig parameter
  events: trigger input FUNCTION_CALL_EVENT
function TOP  = fcn(detentGain_Left, MedusaPremixConfig)
%#codegen
% Checks if the parameter satisfies dimensionality requirements
if(detentGain_Left.Size(1) ~= MedusaPremixConfig.LR_out || detentGain_Left.Size(2) ~= MedusaPremixConfig.LR_in)
    TranslateError('The parameter ''medusa_premix_left_detent'' must be a matrix consisting of %d rows and %d columns.', MedusaPremixConfig.LR_out, MedusaPremixConfig.LR_in);
end

% Checks if the parameter values follow bound requirements
checkValues = (detentGain_Left.Value < 0);    
if(sum(sum(checkValues)))       % Results in 0 if all values in the matrix respect the bound requirements
    TranslateError('The weights in ''medusa_premix_left_detent'' must be greater than or equal to 0.');
end

TOP = detentGain_Left.Value;

end

== matlab function MedusaPremix/PremixWithMonoSurround/SLC Tuning/Detent Level Right/Trivial Translation ==
  data: TOP output; detentGain_Right input; MedusaPremixConfig parameter
  events: trigger input FUNCTION_CALL_EVENT
function TOP  = fcn(detentGain_Right, MedusaPremixConfig)
%#codegen
% Checks if the parameter satisfies dimensionality requirements
if(detentGain_Right.Size(1) ~= MedusaPremixConfig.LR_out || detentGain_Right.Size(2) ~= MedusaPremixConfig.LR_in)
    TranslateError('The parameter ''medusa_premix_right_detent'' must be a matrix consisting of %d rows and %d columns.', MedusaPremixConfig.LR_out, MedusaPremixConfig.LR_in);
end

% Checks if the parameter values follow bound requirements
checkValues = (detentGain_Right.Value < 0);    
if(sum(sum(checkValues)))       % Results in 0 if all values in the matrix respect the bound requirements
    TranslateError('The weights in ''medusa_premix_right_detent'' must be greater than or equal to 0.');
end

TOP = detentGain_Right.Value;

end

== matlab function MedusaPremix/PremixWithMonoSurround/SLC Tuning/Interpolation Method/Trivial Translation ==
  data: TOP output; interpolationMethod input
  events: trigger input FUNCTION_CALL_EVENT
function TOP  = fcn(interpolationMethod)
%#codegen
% Checks if the parameter satisfies dimensionality requirements
if(numel(interpolationMethod.Value) ~= 1)
   TranslateError('The parameter ''medusa_surround_db_interpolation'' must be single dimensional.'); 
end

% Checks if the parameter value follows bound requirements
if((interpolationMethod.Value ~= 0) && (interpolationMethod.Value ~= 1))
   TranslateError('The value of ''medusa_surround_db_interpolation'' must be either 0 (for linear interpolation) or 1 (for dB-linear interpolation).'); 
end

TOP = interpolationMethod.Value;

end

== matlab function MedusaPremix/PremixWithMonoSurround/SLC Tuning/Max Level CS/Trivial Translation ==
  data: TOP output; maxGain_CS input; MedusaPremixConfig parameter
  events: trigger input FUNCTION_CALL_EVENT
function TOP  = fcn(maxGain_CS, MedusaPremixConfig)
%#codegen
% Checks if the parameter satisfies dimensionality requirements
if(maxGain_CS.Size(1) ~= MedusaPremixConfig.CS_out || maxGain_CS.Size(2) ~= MedusaPremixConfig.CS_in)
    TranslateError('The parameter ''medusa_premix_cs_max'' must be a matrix consisting of %d rows and %d columns.', MedusaPremixConfig.CS_out, MedusaPremixConfig.CS_in);
end

% Checks if the parameter values follow bound requirements
checkValues = (maxGain_CS.Value < 0);
if(sum(sum(checkValues)))          % Results in 0 if all values in the matrix respect the bound requirements
    TranslateError('The weights in ''medusa_premix_cs_max'' must be greater than or equal to 0.');
end

TOP = maxGain_CS.Value;

end
